simulink model "adaptive_mpc_controller"  (R2025a)
settings: Solver=FixedStepAuto  StartTime=0.0  StopTime=10.0  RelTol=1e-3
undefined symbols (not defined in the file): A, B, p_btheta, p_bx, p_G, p_g, p_Iw, p_Jp, p_Ke, p_Kt, p_l, p_La, p_M, p_m, p_n, p_r, p_Ra
libraries: simulink x2, mpclib x1, sharedTrackingLibrary x1, eeLuenbergerObserver x1
settings Model: Creator=nopla  LastModifiedBy=nopla
settings OptimizationCC: UseDivisionForNetSlopeComputation=on
settings DebuggingCC: UnderSpecifiedDimensionMsg=warning

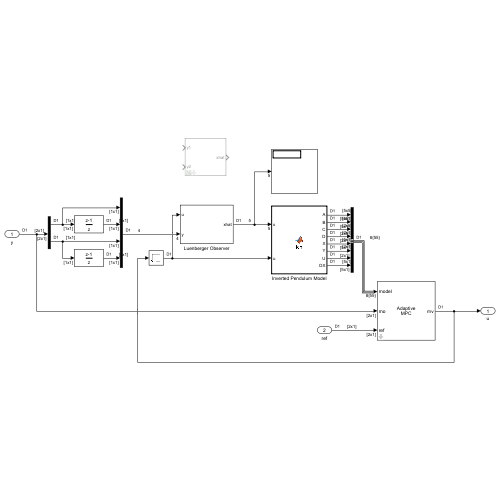
[thumbnail: Simulink's stored preview of the top-level diagram]
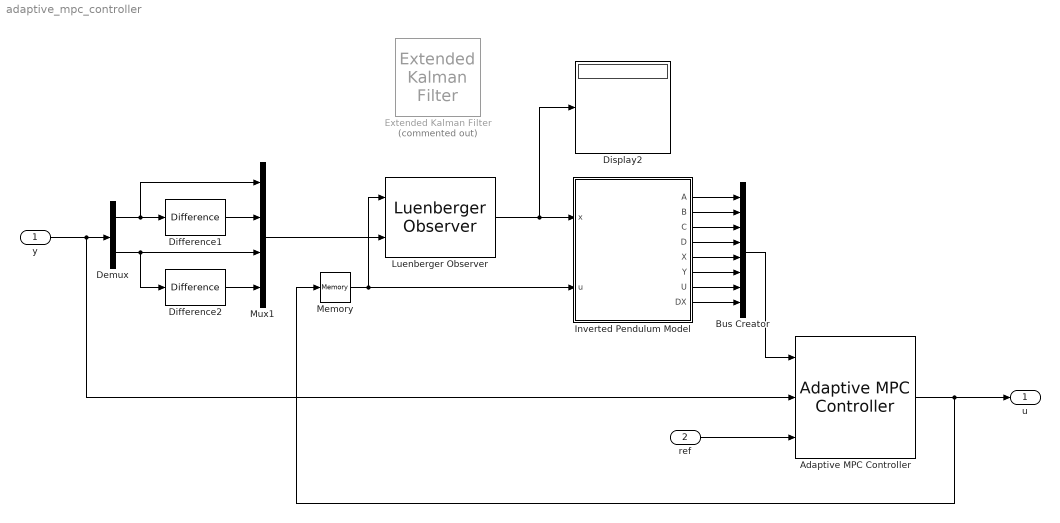
== system adaptive_mpc_controller ==
  y : Inport  PortDimensions=[2 1]
  ref : Inport  Port=2  PortDimensions=[2 1]
  Adaptive MPC Controller : mpclib/Adaptive MPC Controller  SCDEnableBlockLinearizationSpecification=on  mpcobj=ampcobj  enable_value=0  updateMPCinCallerWorkspace=on  md_inport=off  mv_inport=off  uref_inport=off  return_cost=off  return_mvseq=off  return_qpstatus=off  return_xseq=off  return_state=off  return_ovseq=off  state_inport=off  isltv_plant=off  umin_inport=off  umax_inport=off  ymin_inport=off  ymax_inport=off  cc_inport=off  ywt_inport=off  uwt_inport=off  duwt_inport=off  rhoeps_inport=off  pm_inport=off  MaximumP=10  HorizonChoice=FixedHorizon  BlockDataType=double  SampleTimeInherited=off  switch_inport=off
  Bus Creator : BusCreator  Inputs=8
  Demux : Demux  Outputs=2
  Difference1 : simulink/Discrete/Difference  ICPrevInput=0.0  OutMin=[]  OutMax=[]  OutDataType=fixdt(1, 16)  OutScaling=2^-10  DoSatur=off
  Difference2 : simulink/Discrete/Difference  ICPrevInput=0.0  OutMin=[]  OutMax=[]  OutDataType=fixdt(1, 16)  OutScaling=2^-10  DoSatur=off
  Display2 : Display
  Extended Kalman Filter : sharedTrackingLibrary/Extended Kalman Filter  Commented=on  StateTransitionFcn=myStateTransitionFcn  HasStateTransitionJacobianFcn=off  HasAdditiveProcessNoise=Additive  ProcessNoise=1  HasTimeVaryingProcessNoise=off  HasStateTransitionFcnExtraArgument=0  InitialState=0  InitialStateCovariance=1  MeasurementFcn1=myMeasurementFcn  HasMeasurementJacobianFcn1=off  HasMeasurementEnablePort1=off  HasAdditiveMeasurementNoise1=Additive  MeasurementNoise1=1  HasTimeVaryingMeasurementNoise1=off  HasMeasurementFcnExtraArgument1=0  HasMeasurementWrapping1=off  MeasurementFcn2=myMeasurementFcn  HasMeasurementJacobianFcn2=off  HasMeasurementEnablePort2=off  HasAdditiveMeasurementNoise2=Additive  MeasurementNoise2=1  HasTimeVaryingMeasurementNoise2=off  HasMeasurementFcnExtraArgument2=0  HasMeasurementWrapping2=off  MeasurementFcn3=myMeasurementFcn  HasMeasurementJacobianFcn3=off  HasMeasurementEnablePort3=off  HasAdditiveMeasurementNoise3=Additive  MeasurementNoise3=1  HasTimeVaryingMeasurementNoise3=off  HasMeasurementFcnExtraArgument3=0  HasMeasurementWrapping3=off  MeasurementFcn4=myMeasurementFcn  HasMeasurementJacobianFcn4=off  HasMeasurementEnablePort4=off  HasAdditiveMeasurementNoise4=Additive  MeasurementNoise4=1  HasTimeVaryingMeasurementNoise4=off  HasMeasurementFcnExtraArgument4=0  HasMeasurementWrapping4=off  MeasurementFcn5=myMeasurementFcn  HasMeasurementJacobianFcn5=off  HasMeasurementEnablePort5=off  HasAdditiveMeasurementNoise5=Additive  MeasurementNoise5=1  HasTimeVaryingMeasurementNoise5=off  HasMeasurementFcnExtraArgument5=0  HasMeasurementWrapping5=off  EnableMultirate=off  StateTransitionFcnSampleTime=1  MeasurementFcn1SampleTime=1  MeasurementFcn2SampleTime=1  MeasurementFcn3SampleTime=1  MeasurementFcn4SampleTime=1  MeasurementFcn5SampleTime=1  UseCurrentEstimator=on  OutputStateCovariance=off  DataType=double  SampleTime=1  NumberOfMeasurements=2
  Inverted Pendulum Model : MATLAB Function  TreatAsAtomicUnit=on
  Luenberger Observer : eeLuenbergerObserver/Luenberger Observer  StateSpaceType=Continuous-time  Ad=1  Bd=1  Cd=1  Dd=1  A=A  B=B  C=[1 0 0 0 0; 0 1 0 0 0; 0 0 1 0 0; 0 0 0 1 0]  D=[0; 0; 0; 0;]  ObserverDesign=Desired eigenvalues  Ld=1  DesiredEigenvalues=observer_target_eigenvalues  x0=[0; 0; 0; 0; 0]  Tsd=0.1  Ts=0.01
      settings: LibrarySourceBlock=ee_sl_lib/Observers/Luenberger Observer
  Memory : Memory
  Mux1 : Mux
  u : Outport
  wires:
  Inverted Pendulum Model/6(Y) -> Bus Creator/6
  Adaptive MPC Controller/1 -> u/1, Memory/1
  Inverted Pendulum Model/3(C) -> Bus Creator/3
  Inverted Pendulum Model/1(A) -> Bus Creator/1
  Mux1/1 -> Luenberger Observer/2
  Memory/1 -> Luenberger Observer/1, Inverted Pendulum Model/2(u)
  Inverted Pendulum Model/2(B) -> Bus Creator/2
  Inverted Pendulum Model/8(DX) -> Bus Creator/8
  Demux/1 -> Difference1/1, Mux1/1
  Luenberger Observer/1 -> Display2/1, Inverted Pendulum Model/1(x)
  Demux/2 -> Difference2/1, Mux1/3
  Difference1/1 -> Mux1/2
  y/1 -> Adaptive MPC Controller/2, Demux/1
  ref/1 -> Adaptive MPC Controller/3
  Inverted Pendulum Model/4(D) -> Bus Creator/4
  Difference2/1 -> Mux1/4
  Inverted Pendulum Model/7(U) -> Bus Creator/7
  Bus Creator/1 -> Adaptive MPC Controller/1
  Inverted Pendulum Model/5(X) -> Bus Creator/5

== matlab function adaptive_mpc_controller/Inverted Pendulum Model ==
  data: A output; B output; x input; u input; p_M parameter; p_m parameter; p_g parameter; p_l parameter; p_r parameter; p_Iw parameter; p_n parameter; p_G parameter; p_Jp parameter; p_bx parameter; p_btheta parameter; p_Kt parameter; p_Ke parameter; p_Ra parameter; p_La parameter; C output; D output; X output; Y output; U output; DX output
function [A, B, C, D, X, Y, U, DX] = fcn(x, u, p_M, p_m, p_g, p_l, p_r, p_Iw, p_n, p_G, p_Jp, p_bx, p_btheta, p_Kt, p_Ke, p_Ra, p_La)
Ts = 0.01;

[Ac, Bc, Cc, Dc] = pendulum_state_space(p_M, p_m, p_g, p_l, p_r, p_Iw, p_n, p_G, p_Jp, p_bx, p_btheta, p_Kt, p_Ke, p_Ra, p_La);

nx = size(Ac, 1);
nu = size(Bc, 2);
M = expm([[Ac Bc] * Ts; zeros(nu, nx+nu)]);
A = M(1:nx, 1:nx);
B = M(1:nx, nx+1:nx+nu);
C = Cc;
D = Dc;

U = u;
X = x;
Y = C*x + D*u;
DX = A*x + B*u - x;

end
